simulink subsystem "sample_table"  (R2024b)
settings: Solver=VariableStepAuto  StartTime=0.0  StopTime=10.0  RelTol=1e-3
undefined symbols (not defined in the file or in its folder): optimization_time
settings Model: Creator=thatf  LastModifiedBy=thatf

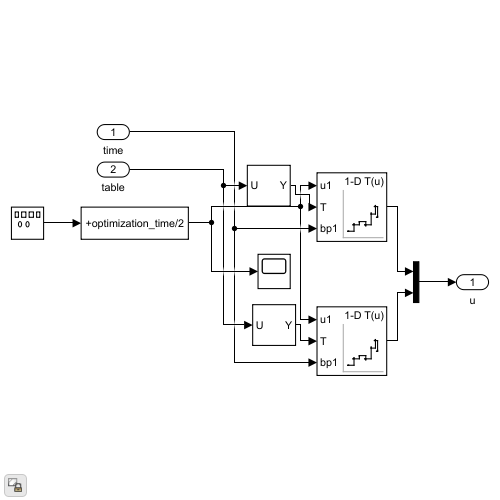
[thumbnail: Simulink's stored preview of the top-level diagram]
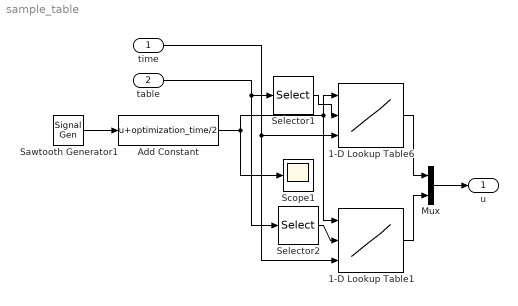
== system sample_table ==
  time : Inport
  table : Inport  Port=2
  1-D Lookup Table1 : Lookup_n-D  NumberOfTableDimensions=1  BreakpointsForDimension1Source=Input port  BreakpointsForDimension1=[-5:5]  TableSource=Input port  Table=tanh([-5:5])  InterpMethod=Flat  InternalRulePriority=Speed  RndMeth=Simplest
      settings: InputPortMap=u0,p221,p5
  1-D Lookup Table6 : Lookup_n-D  NumberOfTableDimensions=1  BreakpointsForDimension1Source=Input port  BreakpointsForDimension1=[-5:5]  TableSource=Input port  Table=tanh([-40:39])  InterpMethod=Flat  InternalRulePriority=Speed  RndMeth=Simplest
      settings: InputPortMap=u0,p221,p5
  Add Constant : Bias  Bias=optimization_time/2  SaturateOnIntegerOverflow=off
  Mux : Mux  Inputs=2
  Sawtooth Generator1 : SignalGenerator  WaveForm=sawtooth  Amplitude=-optimization_time / 2  Frequency=1 / optimization_time
  Scope1 : Scope
  Selector1 : Selector  NumberOfDimensions=2  InputPortWidth=3  IndexOptions=Select all,Index vector (dialog)  Indices=[1],1  OutputSizes=1,1
  Selector2 : Selector  NumberOfDimensions=2  InputPortWidth=3  IndexOptions=Select all,Index vector (dialog)  Indices=[1],2  OutputSizes=1,1
  u : Outport
  wires:
  1-D Lookup Table6/1 -> Mux/1
  Selector1/1 -> 1-D Lookup Table6/2
  Mux/1 -> u/1
  Add Constant/1 -> Scope1/1, 1-D Lookup Table6/1, 1-D Lookup Table1/1
  Sawtooth Generator1/1 -> Add Constant/1
  time/1 -> 1-D Lookup Table6/3, 1-D Lookup Table1/3
  1-D Lookup Table1/1 -> Mux/2
  Selector2/1 -> 1-D Lookup Table1/2
  table/1 -> Selector1/1, Selector2/1
